simulink model "schema_H2016_Quiz1_Gpe1"  (R2014b)
settings: Solver=ode23  StartTime=0.0  StopTime=20  FixedStep=0.001  MaxStep=0.05  RelTol=1e-3
settings Model: Creator=Hugo  LastModifiedBy=Hugo
settings DataIOCC: LimitDataPoints=off
settings DebuggingCC: UnderspecifiedInitializationDetection=Classic  MergeDetectMultiDrivingBlocksExec=none

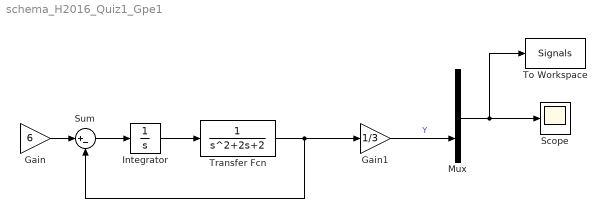
== system schema_H2016_Quiz1_Gpe1 ==
  Gain : Gain  Gain=6
  Gain1 : Gain  Gain=1/3
  Integrator : Integrator
  Mux : Mux  Inputs=2
  Scope : Scope
      settings: ShowLegends=on  SaveName=Datas
  Sum : Sum  Inputs=|+-
  To Workspace : ToWorkspace  VariableName=Signals  SampleTime=-1
  Transfer Fcn : TransferFcn  Denominator=[1 2 2]
  wires:
  Integrator/1 -> Transfer Fcn/1
  Sum/1 -> Integrator/1
  ? -> Gain/1, Mux/1  "Ref"
  Transfer Fcn/1 -> Gain1/1, Sum/2
  Mux/1 -> To Workspace/1, Scope/1
  Gain/1 -> Sum/1
  Gain1/1 -> Mux/2  "Y"
